simulink model "cegla"  (R2018a)
settings: Solver=VariableStepAuto  StartTime=0.0  StopTime=6*10^-3  RelTol=1e-3
StopFcn:
  | Signal_Logs;
  | Burst_Logs;
  | Gap_Logs;
  | Code_Logs;
undefined symbols (not defined in the file or in its folder): generateHann, generateRandomCodedSequence, generateRandomGapSequence, laplace, m
libraries: dspstat3 x19, dspsrcs4 x7, dspsigops x3, commseqgen3 x2
settings Model: Creator=hp  LastModifiedBy=hp

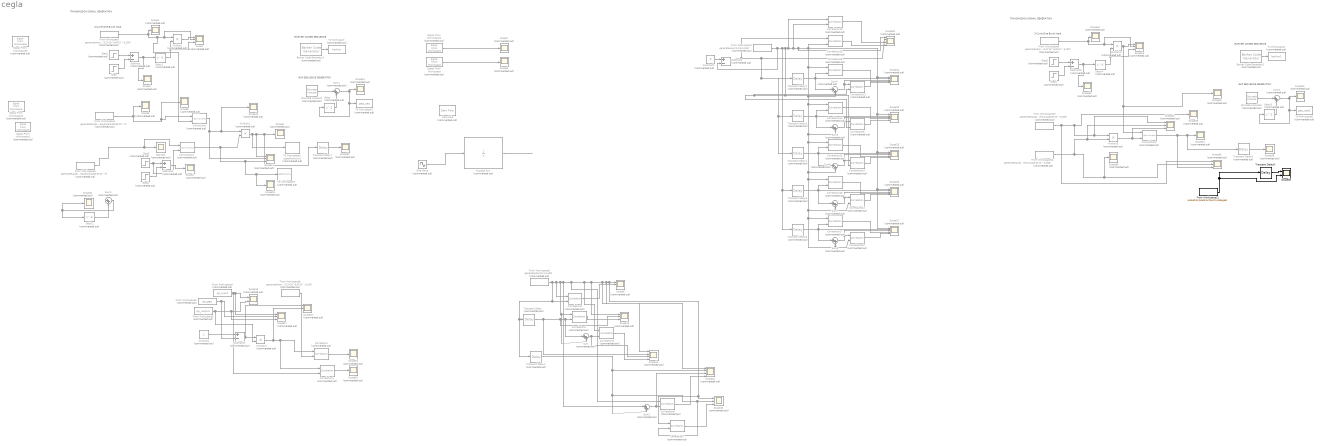
== system cegla ==
  note: BARKER CODED SEQUENCE
  note: 3 Cycle Sine Burst Input
  note: TRANSMISSION SIGNAL GENERATION
  note: GAP SEQUENCE GENERATOR
  note: 3 Cycle Sine Burst Input
  note: GAP SEQUENCE GENERATOR
  note: TRANSMISSION SIGNAL GENERATION
  note: BARKER CODED SEQUENCE
  Barker Code Generator1 : commseqgen3/Barker Code Generator  Commented=on  Length=7  LengthSimulink=7  SampleTime=1  SamplesPerFrame=1  OutputDataType=double  SimulateUsing=Code generation
      settings: SourceProductName=Communications System Toolbox  SourceProductBaseCode=CM
  Barker Code Generator2 : commseqgen3/Barker Code Generator  Commented=on  Length=7  LengthSimulink=7  SampleTime=1  SamplesPerFrame=1  OutputDataType=double  SimulateUsing=Code generation
      settings: SourceProductName=Communications System Toolbox  SourceProductBaseCode=CM
  Constant : Constant  Commented=on
  Constant1 : Constant  Commented=on  Value=0
  Convolution : dspsigops/Convolution  Commented=on  domain=Time  roundingMode=Floor  overflowMode=off  outputDataTypeStr=Inherit: Same as accumulator  outputMin=[]  outputMax=[]  outputLastDataTypeStr=Inherit: Same as accumulator
      settings: SourceProductName=DSP System Toolbox  SourceProductBaseCode=DS
  Convolution1 : dspsigops/Convolution  Commented=on  domain=Time  roundingMode=Floor  overflowMode=off  outputDataTypeStr=Inherit: Same as accumulator  outputMin=[]  outputMax=[]  outputLastDataTypeStr=Inherit: Same as accumulator
      settings: SourceProductName=DSP System Toolbox  SourceProductBaseCode=DS
  Convolution2 : dspsigops/Convolution  Commented=on  domain=Time  roundingMode=Floor  overflowMode=off  outputDataTypeStr=Inherit: Same as accumulator  outputMin=[]  outputMax=[]  outputLastDataTypeStr=Inherit: Same as accumulator
      settings: SourceProductName=DSP System Toolbox  SourceProductBaseCode=DS
  Correlation{,1,3..19} (19 alike) : dspstat3/Correlation  Commented=on  domain=Time  roundingMode=Floor  overflowMode=off  outputDataTypeStr=Inherit: Same as accumulator  outputMin=[]  outputMax=[]  outputLastDataTypeStr=Inherit: Same as accumulator
      settings: SourceProductName=DSP System Toolbox  SourceProductBaseCode=DS
  Delay : Delay  Commented=on
  Delay1 : Delay  Commented=on  DelayLength=0
  Delay2 : Delay  Commented=on  DelayLength=6
  Delay3 : Delay  Commented=on
  Delay4 : Delay  Commented=on  DelayLength=0
  Discrete Impulse1 : dspsrcs4/Discrete  Impulse  Commented=on  Delay=0  SampleTime=1  FrameSample=1  OutputFrames=off  dataType=double  isSigned=on  wordLen=16  udDataType=sfix(16)  fracBitsMode=Best precision  numFracBits=15  OutDataTypeStr=double  LastOutDataTypeStr=double
  Discrete Impulse2 : dspsrcs4/Discrete  Impulse  Commented=on  Delay=0  SampleTime=1  FrameSample=1  OutputFrames=off  dataType=double  isSigned=on  wordLen=16  udDataType=sfix(16)  fracBitsMode=Best precision  numFracBits=15  OutDataTypeStr=double  LastOutDataTypeStr=double
  From Workspace : FromWorkspace  Commented=on  VariableName=generateHann(5,2*10^6,6*10^-3,100)  OutDataTypeStr=double  SampleTime=0.00000001  OutputAfterFinalValue=Setting to zero
  From Workspace1 : FromWorkspace  Commented=on  VariableName=generateRandomCodedSequence(2400,6*10^-3)  OutDataTypeStr=double  SampleTime=0.00000001  Interpolate=off  OutputAfterFinalValue=Setting to zero
  From Workspace10 : FromWorkspace  Commented=on  VariableName=generateRandomCodedSequence(2400,6*10^-3,250)  OutDataTypeStr=double  SampleTime=0.00000001  Interpolate=off  OutputAfterFinalValue=Setting to zero
  From Workspace11 : FromWorkspace  Commented=on  VariableName=generateRandomGapSequence(2400,6*10^-3,250)  OutDataTypeStr=double  SampleTime=0.00000001  Interpolate=off  OutputAfterFinalValue=Setting to zero
  From Workspace12 : FromWorkspace  VariableName=pulseCompression(burst,code,gap)  SampleTime=0
  From Workspace2 : FromWorkspace  Commented=on  VariableName=generateRandomGapSequence(2400,6*10^-3)  OutDataTypeStr=double  SampleTime=0.00000001  Interpolate=off  OutputAfterFinalValue=Setting to zero
  From Workspace3 : FromWorkspace  Commented=on  VariableName=pp_output  SampleTime=0.00000001  Interpolate=off  OutputAfterFinalValue=Setting to zero
  From Workspace4 : FromWorkspace  Commented=on  VariableName=pp_input  SampleTime=0.00000001  Interpolate=off  OutputAfterFinalValue=Setting to zero
  From Workspace5 : FromWorkspace  Commented=on  VariableName=pp_gap  SampleTime=0.00000001  Interpolate=off  OutputAfterFinalValue=Setting to zero
  From Workspace6 : FromWorkspace  Commented=on  VariableName=generateHann(5,1,5,100)  OutDataTypeStr=double  SampleTime=0.00001  OutputAfterFinalValue=Setting to zero
  From Workspace7 : FromWorkspace  Commented=on  VariableName=generateHann(3,0.5,3,100);  OutDataTypeStr=double  SampleTime=0.00001  OutputAfterFinalValue=Setting to zero
  From Workspace8 : FromWorkspace  Commented=on  VariableName=generateHann(5,2*10^6,6*10^-3,100)  OutDataTypeStr=double  SampleTime=0.00000001  OutputAfterFinalValue=Setting to zero
  From Workspace9 : FromWorkspace  Commented=on  VariableName=generateHann(5,2*10^6,6*10^-3,100)  OutDataTypeStr=double  SampleTime=0.00000001  OutputAfterFinalValue=Setting to zero
  "Gap Seq " : Scope  Commented=on
  Multiply{,1..3,5} (5 alike) : Product  Commented=on
  Scope{,9,11,14,17..18,23,31,35,43} (10 alike) : Scope  Commented=on  NumInputPorts=3
  Scope{1..8,10,13,15,19..21,30,32..34,36..38,40,45} (23 alike) : Scope  Commented=on
  Scope12 : Scope  Commented=on  NumInputPorts=4
  Scope16 : Scope  Commented=on  NumInputPorts=2
  Scope22 : Scope  Commented=on  NumInputPorts=4
  Scope{24..27,29} (5 alike) : Scope  Commented=on  NumInputPorts=5
  Scope28 : Scope  Commented=on  NumInputPorts=4
  Scope39 : Scope  NumInputPorts=2
  Signal From Workspace : dspsrcs4/Signal From Workspace  Commented=on  X=laplace(sin(m))  Ts=1  nsamps=1  OutputAfterFinalValue=Setting to zero  ignoreOrWarnInputAndFrameLengths=off  OutputFrames=off
  Signal From Workspace1 : dspsrcs4/Signal From Workspace  Commented=on  X=generateRandomCodedSequence(10)  Ts=1  nsamps=1  OutputAfterFinalValue=Setting to zero  ignoreOrWarnInputAndFrameLengths=off  OutputFrames=off
  Signal From Workspace2 : dspsrcs4/Signal From Workspace  Commented=on  X=generateRandomGapSequence(10)  Ts=1  nsamps=1  OutputAfterFinalValue=Setting to zero  ignoreOrWarnInputAndFrameLengths=off  OutputFrames=off
  Signal From Workspace3 : dspsrcs4/Signal From Workspace  Commented=on  X=generateHann(5,5,10,100)  Ts=.1  nsamps=1  OutputAfterFinalValue=Setting to zero  ignoreOrWarnInputAndFrameLengths=off  OutputFrames=off
  Signal From Workspace4 : dspsrcs4/Signal From Workspace  Commented=on  X=sin(m)  Ts=1  nsamps=1  OutputAfterFinalValue=Setting to zero  ignoreOrWarnInputAndFrameLengths=off  OutputFrames=off
  Sine Wave : Sin  Commented=on  SampleTime=0
  Step : Step  Commented=on  Time=7%/5*10^4
  Step1 : Step  Commented=on  Time=0
  Step2 : Step  Commented=on  Time=7%/5*10^4  VectorParams1D=off
  Step3 : Step  Commented=on  Time=0  VectorParams1D=off
  Step4 : Step  Commented=on  Time=2.5*10^-6
  Step5 : Step  Commented=on  Time=0
  Subtract{,1..4} (5 alike) : Sum  Commented=on  Inputs=+-
  Sum{,1..9} (10 alike) : Sum  Commented=on  Inputs=|++
  To Workspace : ToWorkspace  Commented=on  VariableName=barker  SampleTime=-1
      settings: Save2DSignal=2-D array (concatenate along first dimension)
  To Workspace1 : ToWorkspace  Commented=on  VariableName=gap_seq  SampleTime=-1
  To Workspace2 : ToWorkspace  Commented=on  VariableName=signalfromsimu  SampleTime=-1
      settings: Save2DSignal=2-D array (concatenate along first dimension)
  To Workspace3 : ToWorkspace  Commented=on  VariableName=gapfromsimu  SampleTime=-1
      settings: Save2DSignal=2-D array (concatenate along first dimension)
  To Workspace4 : ToWorkspace  Commented=on  VariableName=barker1  SampleTime=-1
      settings: Save2DSignal=2-D array (concatenate along first dimension)
  To Workspace5 : ToWorkspace  Commented=on  VariableName=gap_seq1  SampleTime=-1
  Transfer Fcn : TransferFcn  Commented=on  Numerator=1  Denominator=[1,0]
  Transport Delay : TransportDelay  Commented=on
  Transport Delay1 : TransportDelay  Commented=on  DelayTime=2
  Transport Delay2 : TransportDelay  Commented=on  DelayTime=0.5
  Transport Delay3 : TransportDelay  Commented=on  DelayTime=2
  Transport Delay4 : TransportDelay  Commented=on  DelayTime=3
  Transport Delay5 : TransportDelay  Commented=on  DelayTime=4
  Transport Delay6 : TransportDelay  Commented=on  DelayTime=5
  Transport Delay7 : TransportDelay  Commented=on  DelayTime=10^-4
  Transport Delay8 : TransportDelay  DelayTime=10^-3
  Transport Delay9 : TransportDelay  Commented=on  DelayTime=10^-3
  Zero-Pole : ZeroPole  Commented=on  Poles=[0 -1]
  wires:
  Subtract1/1 -> Scope2/1
  Step/1 -> Subtract/2
  Step2/1 -> Subtract1/2
  Convolution1/1 -> Scope15/1, To Workspace3/1, Scope14/3, Multiply1/2
  Delay2/1 -> Sum2/2
  Multiply1/1 -> To Workspace2/1, Transport Delay7/1, Scope8/1, Scope14/1
  From Workspace/1 -> Convolution/2, Scope/2, Multiply/1, Scope4/1
  Delay1/1 -> Scope/3, Multiply/2
  Subtract/1 -> Delay1/1, Scope1/1
  Discrete Impulse1/1 -> Sum1/1
  Convolution/1 -> Scope14/2, Scope10/1, Multiply1/1
  Sum1/1 -> To Workspace1/1, Delay/1, Scope13/1
  Step3/1 -> Convolution1/2, Subtract1/1
  Barker Code Generator1/1 -> To Workspace/1
  Delay/1 -> Sum1/2
  Sum2/1 -> Scope21/1, Delay2/1
  Step1/1 -> Subtract/1
  From Workspace1/1 -> Convolution/1, Scope6/1, Scope3/1
  Multiply/1 -> Scope/1
  Sine Wave/1 -> Transfer Fcn/1
  Transfer Fcn/1 -> ?
  Signal From Workspace/1 -> Scope5/1
  Signal From Workspace4/1 -> Scope7/1
  From Workspace2/1 -> Convolution1/1, "Gap Seq "/1
  From Workspace4/1 -> Correlation1/2, Scope17/1, Scope16/1
  From Workspace3/1 -> Multiply3/2, Scope17/3, Scope16/2
  Subtract4/1 -> Scope18/1, Multiply3/1
  Constant/1 -> Subtract4/1
  Multiply3/1 -> Scope18/2, Correlation1/1, Correlation/1
  Correlation1/1 -> Scope20/1
  From Workspace5/1 -> Subtract4/2, Scope17/2
  Correlation/1 -> Scope19/1
  Correlation3/1 -> Scope9/2
  Transport Delay/1 -> Scope12/2, Scope11/2, Sum/1, Correlation4/2
  Correlation4/1 -> Scope11/3
  Sum/1 -> Scope12/3, Correlation5/2
  Correlation5/1 -> Scope12/4
  From Workspace6/1 -> Transport Delay1/1, Transport Delay/1, Correlation3/2, Correlation3/1, Sum3/1, Correlation6/1, Correlation5/1, Scope12/1, Scope22/1, Correlation7/1, Scope23/1, Scope9/1, Scope11/1, Sum/2, Correlation4/1
  Sum3/1 -> Scope22/3, Correlation6/2
  Transport Delay1/1 -> Scope22/2, Correlation7/2, Scope23/2, Sum3/2
  Correlation6/1 -> Scope22/4
  Correlation7/1 -> Scope23/3
  Transport Delay2/1 -> Scope24/2, Sum4/1, Correlation8/2
  Transport Delay3/1 -> Scope29/2, Correlation14/2, Sum5/1
  Transport Delay4/1 -> Scope25/2, Sum6/1, Correlation15/2
  Transport Delay5/1 -> Correlation16/2, Scope26/2, Sum7/1
  Transport Delay6/1 -> Correlation17/2, Scope27/2, Sum8/1
  Sum4/1 -> Scope24/3, Correlation13/1
  Sum5/1 -> Scope29/3, Correlation9/1
  Sum6/1 -> Scope25/3, Correlation10/1
  Sum7/1 -> Scope26/3, Correlation11/1
  Sum8/1 -> Scope27/3, Correlation12/1
  Correlation8/1 -> Scope24/4
  Correlation13/1 -> Scope24/5
  Correlation14/1 -> Scope29/4
  Correlation9/1 -> Scope29/5
  Correlation15/1 -> Scope25/4
  Correlation10/1 -> Scope25/5
  Correlation16/1 -> Scope26/4
  Correlation11/1 -> Scope26/5
  Correlation17/1 -> Scope27/4
  Correlation12/1 -> Scope27/5
  Constant1/1 -> Subtract2/1
  Subtract2/1 -> Correlation18/1, Transport Delay3/1, Transport Delay4/1, Transport Delay2/1, Scope28/2
  Correlation19/1 -> Scope28/3
  Correlation18/1 -> Scope28/4
  From Workspace7/1 -> Subtract2/2, Correlation9/2, Correlation13/2, Correlation10/2, Correlation19/1, Correlation19/2, Scope28/1, Scope27/1, Scope26/1, Scope25/1, Scope29/1, Scope24/1, Sum4/2, Sum5/2, Sum6/2, Correlation11/2, Sum7/2, Sum8/2, Correlation12/2, Correlation17/1, Correlation16/1, Correlation15/1, Correlation14/1, Correlation8/1, Correlation18/2, Transport Delay6/1, Transport Delay5/1
  Transport Delay7/1 -> Scope30/1
  From Workspace8/1 -> Correlation/2
  Transport Delay8/1 -> Scope39/1
  Multiply2/1 -> Scope45/1, Convolution2/1, Scope31/1
  Discrete Impulse2/1 -> Sum9/1
  Delay3/1 -> Sum9/2
  Barker Code Generator2/1 -> To Workspace4/1
  Subtract3/1 -> Delay4/1, Scope32/1
  Delay4/1 -> Scope31/3, Multiply2/2
  Step4/1 -> Subtract3/2
  Step5/1 -> Subtract3/1
  From Workspace10/1 -> Scope35/1, Scope33/1, Scope43/1, Multiply5/1
  From Workspace9/1 -> Scope31/2, Multiply2/1, Scope40/1
  Sum9/1 -> To Workspace5/1, Delay3/1, Scope34/1
  From Workspace11/1 -> Multiply5/2, Scope43/2, Scope35/2, Scope36/1
  Multiply5/1 -> Scope43/3, Convolution2/2
  Transport Delay9/1 -> Scope38/1
  Convolution2/1 -> Transport Delay9/1, Scope37/1, Scope35/3
  From Workspace12/1 -> Scope39/2, Transport Delay8/1
